simulink library "PhdLibrary"  (R2020a)
settings: Solver=VariableStepAuto  StartTime=0.0  StopTime=10.0  RelTol=1e-3
undefined symbols (not defined in the file): A1, A2, Asigma, Atilde1, Atilde2, B, B1, B2, bsigma, C1, CiL, Cmatrix, Csigma, Ctilde1, Dtilde1, Dtilde2, F1, G1, L, L1, LobsiL, magnitude, Masigma, Nasigma, ObsEp, obsSys, P2, R, R1, rho, RMSfrequency, Ro, Smep, T, ueq, x_e, xe
libraries: $bdroot x6, simulink x2, powerlib_meascontrol x1, dspstat3 x1, dspmathops x1
settings Model: Creator=d13go  LastModifiedBy=d13go

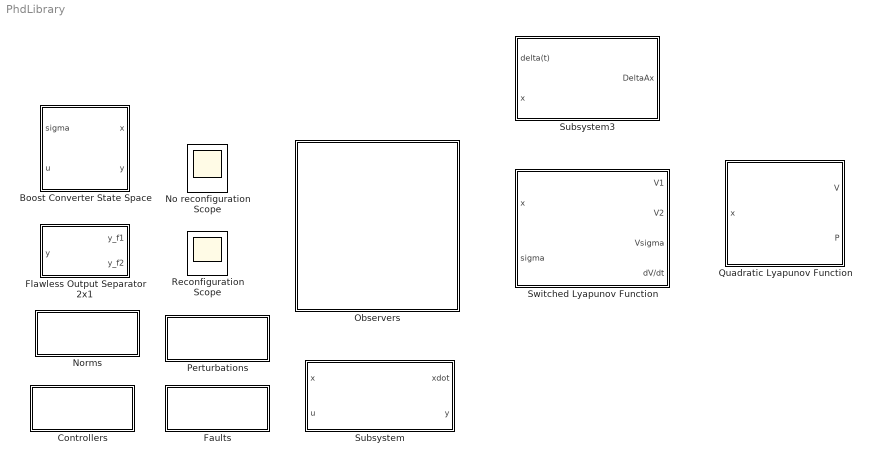
== system PhdLibrary ==
  Boost Converter State Space : Subsystem  mask(Boots State-Space model){A1=A1, A2=A2, B1=B1, R=R, Ro=Ro, Cmatrix=Cmatrix}
      mask prompts: A1 "A1 matrix"; A2 "A2 matrix"; B1 "B matrix"; R "Resistance"; Ro "Output Resistance"; Cmatrix "Output Matrix"
      mask help: Boots State-Space model
      mask Display: disp('Boost')
  Controllers : Subsystem
  Faults : Subsystem
  Flawless Output Separator 2x1 : Subsystem  mask(Flawless Output Separator){Cf1=0, Cf2=0}
      mask prompts: Cf1 "Fault matrix 1"; Cf2 "Fault matrix 2"
      mask help: Separates the 2x1 output
  No reconfiguration Scope : Scope
  Norms : Subsystem
  Observers : Subsystem
  Perturbations : Subsystem
  Quadratic Lyapunov Function : Subsystem  mask{P=P2}
      mask DialogControl DescTextVar Prompt: V = x'Px
      mask Display: disp('Quadratic \nLyapunov \nfunction')
  Reconfiguration Scope : Scope
  Subsystem : Subsystem  mask{A=A1, B=B1, C=C1}
      mask prompts: A "Matrix A"; B "Matrix B"; C "Matrix C"
      mask Display: disp('Static State Space \n xdot = Ax+Bu\n y =Cx')
  Subsystem3 : Subsystem  mask{M=Masigma{1}, N=Nasigma{1}}
      mask prompts: M "M matrix"; N "N matrix"
      mask DialogControl DescTextVar Prompt: Uncertainties matrices of type \DeltaA = delta(t)*MaNa*x(t)
      mask Display: disp('Norm-bounded \n uncertainty')
  Switched Lyapunov Function : Subsystem  mask{P1=obsSys{3}.P{1}, P2=obsSys{3}.P{2}}
      mask Display: disp('Switched \n Lyapunov \n Function\n 2-Subsystems')

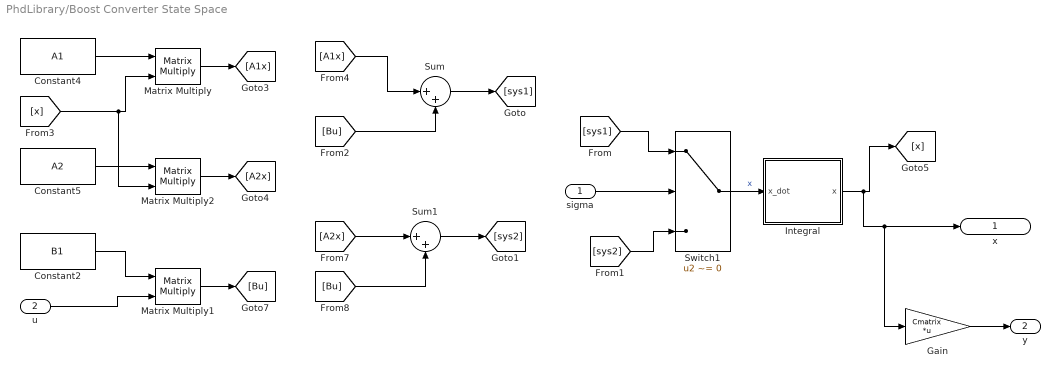
== system PhdLibrary/Boost Converter State Space ==
  sigma : Inport
  u : Inport  Port=2
  Constant2 : Constant  Value=B1  VectorParams1D=off
  Constant4 : Constant  Value=A1  VectorParams1D=off
  Constant5 : Constant  Value=A2  VectorParams1D=off
  Gain : Gain  Gain=Cmatrix  Multiplication=Matrix(K*u)
  Integral : Subsystem
  Matrix Multiply : Product  Multiplication=Matrix(*)
  Matrix Multiply1 : Product  Multiplication=Matrix(*)
  Matrix Multiply2 : Product  Multiplication=Matrix(*)
  Sum : Sum  Inputs=|++
  Sum1 : Sum  Inputs=|++
  Switch1 : Switch  Criteria=u2 ~= 0
  x : Outport
  y : Outport  Port=2
  wires:
  [A1x] -> Sum/1
  [x] -> Matrix Multiply2/2, Matrix Multiply/2
  [Bu] -> Sum1/2
  [Bu] -> Sum/2
  Constant5/1 -> Matrix Multiply2/1
  Constant4/1 -> Matrix Multiply/1
  Matrix Multiply2/1 -> [A2x]
  [sys1] -> Switch1/1
  Matrix Multiply/1 -> [A1x]
  Sum/1 -> [sys1]
  Sum1/1 -> [sys2]
  [sys2] -> Switch1/3
  Switch1/1 -> Integral/1(x_dot)  "x"
  [A2x] -> Sum1/1
  sigma/1 -> Switch1/2
  Constant2/1 -> Matrix Multiply1/1
  Matrix Multiply1/1 -> [Bu]
  u/1 -> Matrix Multiply1/2
  Integral/1(x) -> Gain/1, x/1, [x]
  Gain/1 -> y/1

== system PhdLibrary/Controllers ==
  Equilibrium Point : Subsystem  mask(Equilibrium point){R=0, Ro=0}
      mask prompts: R "Resistance"; Ro "Output resistance"
      mask help: Calculates the equilibrium point
  Integral Sliding Mode Controller : Subsystem  mask(Sliding mode controller){KiVc=2.3, KVc=0.2, ueq=ueq, Smep=Smep, KiL=2, Freq=7000}
      mask prompts: KiVc "Integral voltage gain"; KVc "Voltage gain"; ueq "Equilibrium signal"; Smep "Surface limit layer"; KiL "Current gain"; Freq "Frequency"
      mask help: Sliding mode controller with integral for boost converter
  Limit Layer : $bdroot/Controllers/Integral Sliding  Mode Controller/SlidingSurface  Smep=Smep
  Subsystem1 : Subsystem  mask{A=A1, B=B1}
      mask prompts: A "A matrx"; B "B matrix"
      mask Display: disp("Switching \n Signal \n 1-subsystem");
  Switched Affine Control : Subsystem  mask(Switched linear affine Controler){A1=0, A2=0, B1=0, B2=0, P=0}
      mask prompts: A1 "System matrix 1:"; A2 "System matrix 2:"; B1 "Input matrix 1:"; B2 "Input matrix 2:"; P "Gain matrix:"
      mask help: Controller to generate a switching law according to the equilibrium point xe

== system PhdLibrary/Faults ==
  Fault Detector : Subsystem  mask(Fault detector){Jth=0}
      mask prompts: Jth "Residual threshold"
      mask help: Generates alarm (1) if J > Jth
  Loss of sensor Generator : Subsystem  mask(Loss of sensor signal fault generator){}
      mask help: Loss of signal fault
  Noise Fault Generator : Subsystem  mask(Noise fault generator){}
      mask help: Generates noise in the desired sensor
  Offset Fault Generator : Subsystem  mask(Step faults){s1gain=20, s2gain=20}
      mask prompts: s1gain "Sensor 1 fault gain:"; s2gain "Sensor 2 fault gain:"
      mask help: Configure a step fault
  Sensor Gain Fault Generator : Subsystem  mask(Sensor gain fault generator){s1gain=0, s2gain=0}
      mask prompts: s1gain "Sensor 1 gain fault:"; s2gain "Sensor 2 gain fault:"
      mask help: Generates a gain fault in each sensor

== system PhdLibrary/Flawless Output Separator 2x1 ==
  y : Inport
  Matrizes A1 : Constant  Value=Cf2  VectorParams1D=off
  Matrizes A2 : Constant  Value=Cf1  VectorParams1D=off
  Product : Product  Multiplication=Matrix(*)
  Product1 : Product  Multiplication=Matrix(*)
  y_f1 : Outport
  y_f2 : Outport  Port=2
  wires:
  y/1 -> Product1/2, Product/2
  Matrizes A2/1 -> Product/1
  Matrizes A1/1 -> Product1/1
  Product/1 -> y_f1/1
  Product1/1 -> y_f2/1

== system PhdLibrary/Norms ==
  Norm : Subsystem
      mask DialogControl DescTextVar Prompt: Norm of a vector corresponding to ||u|| or \sqrt(u'u)
      mask Display: disp('Norm')
  Residual Evaluation RMS : Subsystem  mask{RMSfrequency=RMSfrequency/10}
      mask prompts: RMSfrequency "Windows length:"
      mask help: RMS generator for two dimensios

== system PhdLibrary/Observers ==
  Augmented Error Generator : Subsystem  mask{Cmatrix=Cmatrix, Ctilde1=Ctilde1}
      mask prompts: Cmatrix "Output Matrix"; Ctilde1 "Output matrix augmented:"
  FDSMOSLS : Subsystem  mask(Sliding mode observer){G=G1, F=F1, Atilde1=Atilde1, Atilde2=Atilde2, Dtilde1=Dtilde1, Dtilde2=Dtilde2, Ctilde1=Ctilde1, rho=rho}
      mask prompts: G "G matrix"; F "F matrix"; Atilde1 "A1 matrix augmented"; Atilde2 "A2 matrix augmented"; Dtilde1 "D1 matrix augmented"; Dtilde2 "D2 matrix augmented"; Ctilde1 "C1 matrix augmented"; rho "Sliding surface coefficient (rho)"
      mask help: Sligin mode observer for fault detection in switched affine linear systems
      mask Help: Enter the system matrices and the observer gains
      mask Display: disp('\dot{x} = Ax + b \\ y = Cx','texmode','on');
  ROSLSO 2 Subsystems : Subsystem  mask(ROSLSO){B1=0, B2=0, T=0, F1=0, F2=0, L1=0, L2=0, Q=0, z0=0}
      mask prompts: B1 "Input matrix system 1:"; B2 "Input matrix system 2:"; T "Input gain matrix:"; F1 "Observer matrix system 1:"; F2 "Observer matrix system 2:"; L1 "Output gain matrix system 1:"; L2 "Output gain matrix system 2:"; Q "Weight matrix"; z0 "Initial conditions:"
      mask help:
      | Reduced Order Switched Linear Systems Observer
      | Estimates only the unmensured variables and concatenate with output
  Reduced Order Observer : Subsystem  mask(Reduced order observer for linear systems){F=0, L=0, T=0, B=0, Q=0, z0=0}
      mask prompts: F "Observer gain matrix:"; L "Output gain matrix:"; T "Input gain matrix:"; B "Input matrix:"; Q "Weight matrix:"; z0 "Intial conditions"
      mask help:
      | Generates the estimation of unmeasured outputs with a concatenation of the output
      | z is the output unmeasured
      | x hat is the whole state estimation
  Reduced Order Derivate Z : Subsystem  mask(Reduced Order Observer Derivate Z){F=0, L=L, T=T, B=B}
      mask prompts: F "Observer gain matrix:"; L "Output gain matrix:"; T "Input gain matrix:"; B "Input matrix:"
      mask help: Reduced Order Observer Derivate Z generates just zdot, without feedbak
  Residual Generator : Subsystem  mask{A=A1, B=B1, L=L1, C=C1, R=R1}
      mask prompts: A "Matrix A"; B "Matrix B"; L "Matrix L"; C "Matrix C"; R "Matrix R"
      mask DialogControl DescTextVar Prompt: dxhat/dt = A*xhat + B*u + L*(y-yhat)
      mask DialogControl Control2 Prompt: yhat = C*xhat
      mask Display: disp('Luenberger Residual \n Generator')
  SMOSLS : Subsystem  mask(Sliding mode observer for Switched linear affine systems){A1=A1, A2=A2, B1=B1, B2=B2, C1=CiL, L=LobsiL, Smep=ObsEp, yhat0=0, x0=[0;0]}
      mask prompts: A1 "System matrix 1:"; A2 "System matrix 2:"; B1 "Input matrix 1:"; B2 "Input matrix 2:"; C1 "Output matrix 1:"; L "Observer gain:"; Smep "Limit layer:"; yhat0 "Output initial condition:"; x0 "Observer initial condition:"
      mask help: Full order observer that estimates the full state of a switched affine linear system
  Switched Residual Generator : Subsystem  mask(Boots State-Space model){A1=obsSys{2}.Asigma{1,1}, B1=obsSys{2}.bsigma{1,1}, L1=obsSys{2}.Lsigma{1,1}, C1=obsSys{2}.Csigma{1,1}, R1=obsSys{2}.Rsigma{1,1}, A2=obsSys{2}.Asigma{1,2}, B2=obsSys{2}.bsigma{1,1}, C2=obsSys{2}.Csigma{1,1}, L2=obsSys{2}.Lsigma{1,2}, R2=obsSys{2}.Rsigma{1,2}}
      mask prompts: A1 "A1 matrix"; B1 "B1 matrix"; L1 "L1 matrix"; C1 "C1 Matrix"; R1 "R1 matrix"; A2 "A2 matrix"; B2 "B2 matrix"; C2 "C2 matrix"; L2 "L2 matrix"; R2 "R2 matrix"
      mask help: Boots State-Space model
      mask DialogControl DescTextVar Prompt: dxhat/dt = A(sigma)*xhat+B(sigma)*u + L(sigma)*(y-yhat)
      mask DialogControl Control2 Prompt: yhat = C(sigma)*xhat
      mask DialogControl Control3 Prompt: r = R(sigma)*(y-yhat)
      mask DialogControl Subsystem1 Prompt: Subsystem 1
      mask DialogControl Subsystem2 Prompt: Subsytem 2
      mask Display: disp('Switched Luenberger \n Residual Generator \n 2-Subsystems')
  Uncertain Cuk : Subsystem  mask{A1=Asigma{1}, B1=bsigma{1}, C1=Csigma{1}, A2=Asigma{2}, B2=bsigma{2}, C2=Csigma{2}}
      mask prompts: A1 "Matrix A"; B1 "Matrix B"; C1 "Matrix C"; A2 "Matrix A"; B2 "Matrix B"; C2 "Matrix C"
      mask DialogControl DescTextVar Prompt: dx/dt = A(sigma)x+ B(sigma)u + wx(sigma,x,u,t)
      mask DialogControl Control2 Prompt: y = C(sigma)x + wy(sigma,x,u,t)
      mask DialogControl Container3 Prompt: Subsystem 1
      mask DialogControl Container4 Prompt: Subsystem 2
      mask Display: disp('Switched Perturbed State Space \n 2-Subsystems')

== system PhdLibrary/Perturbations ==
  Step Perturbation : Subsystem  mask(Step Perturbation){SignalSwitch=0, InitialMagnitude=0, InitialTime=0, Magnitude=0, Duration=0}
      mask prompts: SignalSwitch "Type of perturbation:"; InitialMagnitude "Initial magnitude"; InitialTime "Initial time:"; Duration "Duration (if transient):"
      mask help:
      | Insert a  persistent or transient step perturbation in the system with given magnitude and time.
      | Type of perturbation: 1 if persistent, 0 if transient
  Transient Step Perturbation : Subsystem  mask(Step perturbation){InitialTime=0.5, Duration=0.1, InitialMagnitude=0, Magnitude=1}
      mask prompts: InitialTime "Initial time:"; InitialMagnitude "Initial magnitude:"
      mask help: Insert a step perturbation with time delta

== system PhdLibrary/Quadratic Lyapunov Function ==
  x : Inport
  Constant : Constant  Value=P
  Gain : Gain  Gain=P  Multiplication=Matrix(u*K)
  Matrix Multiply : Product  Multiplication=Matrix(*)
  Transpose : Math  Operator=transpose  SaturateOnIntegerOverflow=on
  V : Outport
  P : Outport  Port=2
  wires:
  x/1 -> Matrix Multiply/2, Transpose/1
  Matrix Multiply/1 -> V/1
  Transpose/1 -> Gain/1
  Constant/1 -> P/1
  Gain/1 -> Matrix Multiply/1

== system PhdLibrary/Subsystem ==
  x : Inport
  u : Inport  Port=2
  Gain : Gain  Gain=B  Multiplication=Matrix(K*u) (u vector)
  Gain1 : Gain  Gain=A  Multiplication=Matrix(K*u) (u vector)
  Gain2 : Gain  Gain=C  Multiplication=Matrix(K*u) (u vector)
  Sum : Sum  Inputs=|++
  xdot : Outport
  y : Outport  Port=2
  wires:
  u/1 -> Gain/1
  x/1 -> Gain2/1, Gain1/1
  Gain1/1 -> Sum/1
  Gain/1 -> Sum/2
  Sum/1 -> xdot/1
  Gain2/1 -> y/1

== system PhdLibrary/Subsystem3 ==
  delta(t) : Inport
  x : Inport  Port=2
  Constant : Constant  Value=M
  Constant1 : Constant  Value=N
  Matrix Multiply1 : Product
  Matrix Multiply2 : Product  Multiplication=Matrix(*)
  Matrix Multiply3 : Product  Multiplication=Matrix(*)
  DeltaAx : Outport
  wires:
  Constant/1 -> Matrix Multiply3/1
  Constant1/1 -> Matrix Multiply3/2
  Matrix Multiply3/1 -> Matrix Multiply1/2
  delta(t)/1 -> Matrix Multiply1/1
  Matrix Multiply1/1 -> Matrix Multiply2/1
  x/1 -> Matrix Multiply2/2
  Matrix Multiply2/1 -> DeltaAx/1

== system PhdLibrary/Switched Lyapunov Function ==
  x : Inport
  sigma : Inport  Port=2
  Derivative : Derivative
  Quadratic Lyapunov Function2 : $bdroot/Quadratic Lyapunov Function  P=P2
  Quadratic Lyapunov Function3 : $bdroot/Quadratic Lyapunov Function  P=P2
  Switch : Switch  Threshold=2
  V1 : Outport
  V2 : Outport  Port=2
  Vsigma : Outport  Port=3
  dV/dt : Outport  Port=4
  wires:
  Quadratic Lyapunov Function3/1 -> Switch/1, V2/1
  Quadratic Lyapunov Function2/1 -> Switch/3, V1/1
  x/1 -> Quadratic Lyapunov Function3/1, Quadratic Lyapunov Function2/1
  sigma/1 -> Switch/2
  Switch/1 -> Derivative/1, Vsigma/1
  Derivative/1 -> dV/dt/1

== system PhdLibrary/Boost Converter State Space/Integral ==
  x_dot : Inport
  Ground : Ground
  Ground1 : Ground
  IC : InitialCondition  Value=[0;0]
  Integrator1 : Integrator  InitialConditionSource=external  InitialCondition=[-x_e; 0; 0]
  Mux : Mux  Inputs=2
  x : Outport
  wires:
  x_dot/1 -> Integrator1/1
  Integrator1/1 -> x/1
  IC/1 -> Integrator1/2
  Ground1/1 -> Mux/2
  Ground/1 -> Mux/1
  Mux/1 -> IC/1

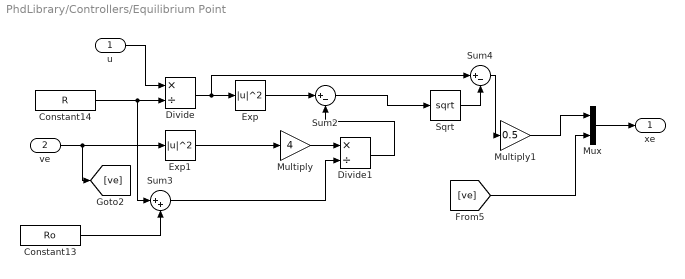
== system PhdLibrary/Controllers/Equilibrium Point ==
  u : Inport
  ve : Inport  Port=2
  Constant13 : Constant  Value=Ro  VectorParams1D=off
  Constant14 : Constant  Value=R  VectorParams1D=off
  Divide : Product  Inputs=*/
  Divide1 : Product  Inputs=*/
  Exp : Math  Operator=magnitude^2  SaturateOnIntegerOverflow=on
  Exp1 : Math  Operator=magnitude^2  SaturateOnIntegerOverflow=on
  Multiply : Gain  Gain=4
  Multiply1 : Gain  Gain=0.5
  Mux : Mux  Inputs=2
  Sqrt : Sqrt  SaturateOnIntegerOverflow=on
  Sum2 : Sum  Inputs=|+-
  Sum3 : Sum  Inputs=|++
  Sum4 : Sum  Inputs=|+-
  xe : Outport
  wires:
  Divide/1 -> Sum4/1, Exp/1
  Sum3/1 -> Divide1/2
  Sum4/1 -> Multiply1/1
  [ve] -> Mux/2
  Multiply/1 -> Divide1/1
  u/1 -> Divide/1
  Constant13/1 -> Sum3/2
  Sqrt/1 -> Sum4/2
  ve/1 -> [ve], Exp1/1
  Exp/1 -> Sum2/1
  Multiply1/1 -> Mux/1
  Mux/1 -> xe/1
  Sum2/1 -> Sqrt/1
  Constant14/1 -> Sum3/1, Divide/2
  Divide1/1 -> Sum2/2
  Exp1/1 -> Multiply/1

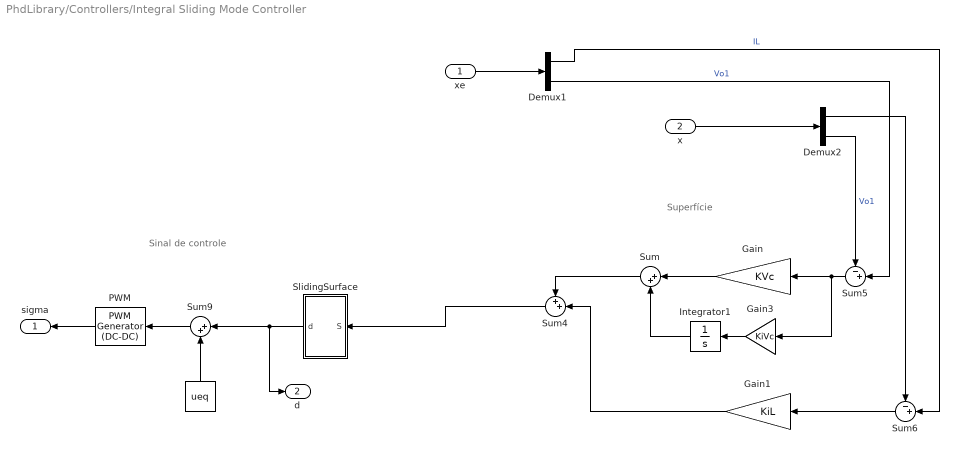
== system PhdLibrary/Controllers/Integral Sliding Mode Controller ==
  note: Sinal de controle
  note: Superfície
  xe : Inport
  x : Inport  Port=2
  "    " : Constant  Value=ueq
  Demux1 : Demux  Outputs=2
  Demux2 : Demux  Outputs=2
  Gain : Gain  Gain=KVc
  Gain1 : Gain  Gain=KiL
  Gain3 : Gain  Gain=KiVc
  Integrator1 : Integrator
  PWM : powerlib_meascontrol/Pulse & Signal Generators/PWM Generator (DC-DC)  Fsw=Freq  Ts=0
  SlidingSurface : Subsystem  mask(Sliding mode limit layer){Smep=Smep}
      mask prompts: Smep "Limit layer value"
      mask help: Define a limit layer for the sliding mode signal
      mask DialogControl ParametersGroupVar Prompt: Parameters
  Sum : Sum  Inputs=|++
  Sum4 : Sum  Inputs=++|
  Sum5 : Sum  Inputs=-+|
  Sum6 : Sum  Inputs=-+|
  Sum9 : Sum  Inputs=|++
  sigma : Outport
  d : Outport  Port=2
  wires:
  Demux1/1 -> Sum6/2  "IL"
  PWM/1 -> sigma/1
  Demux2/2 -> Sum5/1  "Vo1"
  "    "/1 -> Sum9/2
  Sum5/1 -> Gain3/1, Gain/1
  Sum9/1 -> PWM/1
  Demux1/2 -> Sum5/2  "Vo1"
  Demux2/1 -> Sum6/1
  x/1 -> Demux2/1
  Gain1/1 -> Sum4/2
  Gain/1 -> Sum/1
  Sum/1 -> Sum4/1
  SlidingSurface/1(d) -> d/1, Sum9/1
  Sum6/1 -> Gain1/1
  Gain3/1 -> Integrator1/1
  Sum4/1 -> SlidingSurface/1(S)
  Integrator1/1 -> Sum/2
  xe/1 -> Demux1/1

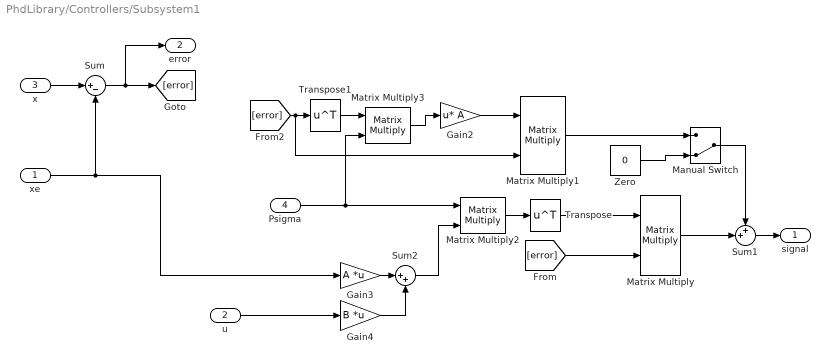
== system PhdLibrary/Controllers/Subsystem1 ==
  xe : Inport
  u : Inport  Port=2
  x : Inport  Port=3
  Psigma : Inport  Port=4
  Gain2 : Gain  Gain=A  Multiplication=Matrix(u*K)
  Gain3 : Gain  Gain=A  Multiplication=Matrix(K*u)
  Gain4 : Gain  Gain=B  Multiplication=Matrix(K*u)
  Manual Switch : ManualSwitch  CurrentSetting=0
  Matrix Multiply{,1..3} (4 alike) : Product  Multiplication=Matrix(*)
  Sum : Sum  Inputs=|+-
  Sum1 : Sum  Inputs=++|
  Sum2 : Sum  Inputs=|++
  Transpose : Math  Operator=transpose  SaturateOnIntegerOverflow=on
  Transpose1 : Math  Operator=transpose  SaturateOnIntegerOverflow=on
  Zero : Constant  Value=0  OutDataTypeStr=Inherit: Inherit via back propagation
  signal : Outport
  error : Outport  Port=2
  wires:
  Matrix Multiply2/1 -> Transpose/1
  Gain3/1 -> Sum2/1
  u/1 -> Gain4/1
  Gain4/1 -> Sum2/2
  x/1 -> Sum/1
  Sum/1 -> error/1, [error]
  [error] -> Matrix Multiply/2
  Transpose/1 -> Matrix Multiply/1
  Matrix Multiply/1 -> Sum1/2
  Sum1/1 -> signal/1
  Gain2/1 -> Matrix Multiply1/1
  [error] -> Matrix Multiply1/2, Transpose1/1
  xe/1 -> Sum/2, Gain3/1
  Psigma/1 -> Matrix Multiply3/2, Matrix Multiply2/1
  Matrix Multiply3/1 -> Gain2/1
  Transpose1/1 -> Matrix Multiply3/1
  Sum2/1 -> Matrix Multiply2/2
  Matrix Multiply1/1 -> Manual Switch/1
  Manual Switch/1 -> Sum1/1
  Zero/1 -> Manual Switch/2

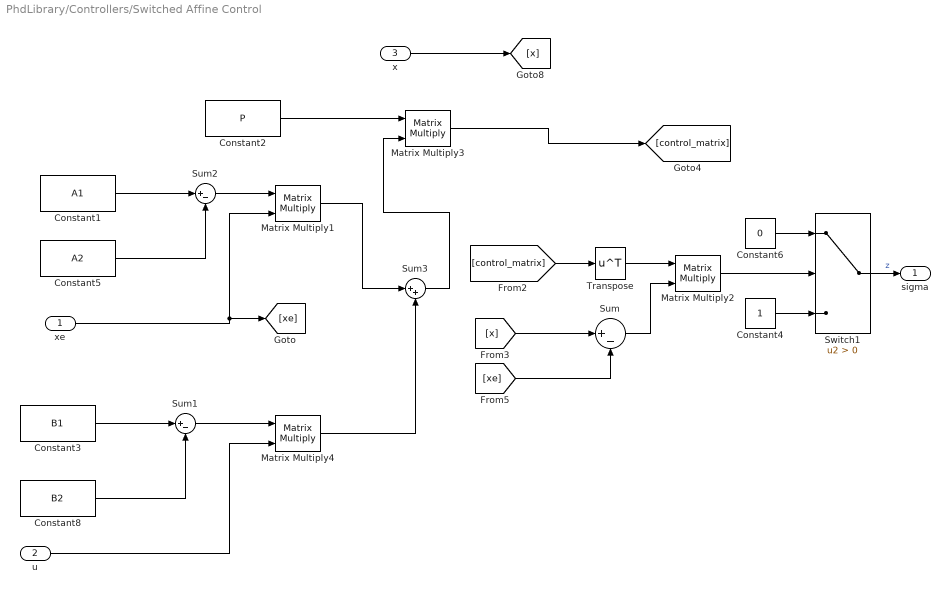
== system PhdLibrary/Controllers/Switched Affine Control ==
  xe : Inport
  u : Inport  Port=2
  x : Inport  Port=3
  Constant1 : Constant  Value=A1  VectorParams1D=off
  Constant2 : Constant  Value=P  VectorParams1D=off
  Constant3 : Constant  Value=B1  VectorParams1D=off
  Constant4 : Constant
  Constant5 : Constant  Value=A2  VectorParams1D=off
  Constant6 : Constant  Value=0
  Constant8 : Constant  Value=B2  VectorParams1D=off
  Matrix Multiply{1..4} (4 alike) : Product  Multiplication=Matrix(*)
  Sum : Sum  Inputs=|+-
  Sum1 : Sum  Inputs=|+-
  Sum2 : Sum  Inputs=|+-
  Sum3 : Sum  Inputs=|++
  Switch1 : Switch  Criteria=u2 > Threshold
  Transpose : Math  Operator=transpose  SaturateOnIntegerOverflow=on
  sigma : Outport
  wires:
  Constant5/1 -> Sum2/2
  Matrix Multiply2/1 -> Switch1/2
  [control_matrix] -> Transpose/1
  Constant1/1 -> Sum2/1
  Constant6/1 -> Switch1/1
  Sum/1 -> Matrix Multiply2/2
  [xe] -> Sum/2
  [x] -> Sum/1
  Constant4/1 -> Switch1/3
  x/1 -> [x]
  Transpose/1 -> Matrix Multiply2/1
  Constant2/1 -> Matrix Multiply3/1
  Switch1/1 -> sigma/1  "z"
  Constant3/1 -> Sum1/1
  Constant8/1 -> Sum1/2
  Sum2/1 -> Matrix Multiply1/1
  Sum1/1 -> Matrix Multiply4/1
  u/1 -> Matrix Multiply4/2
  xe/1 -> [xe], Matrix Multiply1/2
  Matrix Multiply1/1 -> Sum3/1
  Matrix Multiply4/1 -> Sum3/2
  Sum3/1 -> Matrix Multiply3/2
  Matrix Multiply3/1 -> [control_matrix]

== system PhdLibrary/Faults/Fault Detector ==
  Residual : Inport
  Constant10 : Constant
  Constant9 : Constant  Value=0
  Fault Detecition : Switch  Criteria=u2 > Threshold  Threshold=Jth  ZeroCross=off
  Alarm : Outport
  wires:
  Constant9/1 -> Fault Detecition/3
  Constant10/1 -> Fault Detecition/1
  Fault Detecition/1 -> Alarm/1
  Residual/1 -> Fault Detecition/2

== system PhdLibrary/Faults/Loss of sensor Generator ==
  y : Inport
  faultType : Inport  Port=2
  Constant4 : Constant  Value=[1 0;0 1]  VectorParams1D=off
  Constant7 : Constant  Value=[0 0;0 1]  VectorParams1D=off
  Constant8 : Constant  Value=[1 0;0 0]  VectorParams1D=off
  Fault Switch : MultiPortSwitch  DataPortOrder=Zero-based contiguous  DataPortForDefault=Additional data port  zeroidx=on
  Matrix Multiply : Product  Multiplication=Matrix(*)
  yfault : Outport
  wires:
  Constant7/1 -> Fault Switch/3
  Constant4/1 -> Fault Switch/5, Fault Switch/2
  Constant8/1 -> Fault Switch/4
  Fault Switch/1 -> Matrix Multiply/1
  faultType/1 -> Fault Switch/1
  Matrix Multiply/1 -> yfault/1
  y/1 -> Matrix Multiply/2

== system PhdLibrary/Faults/Noise Fault Generator ==
  y : Inport
  faultType : Inport  Port=2
  Band-Limited White Noise1 : simulink/Sources/Band-Limited White Noise  Cov=[0.1]  Ts=0.1  seed=[23341]  VectorParams1D=off
  Constant2 : Constant  Value=[0 0;0 0]  VectorParams1D=off
  Constant5 : Constant  Value=[1 0;0 0]  VectorParams1D=off
  Constant6 : Constant  Value=[0 0;0 1]  VectorParams1D=off
  Matrix Multiply : Product  Multiplication=Matrix(*)
  Noise Fault Switch : MultiPortSwitch  DataPortOrder=Zero-based contiguous  DataPortForDefault=Additional data port  zeroidx=on
  Sum1 : Sum  Inputs=|++
  yfault : Outport
  wires:
  faultType/1 -> Noise Fault Switch/1
  Constant5/1 -> Noise Fault Switch/3
  Constant6/1 -> Noise Fault Switch/4
  Band-Limited White Noise1/1 -> Matrix Multiply/2
  Noise Fault Switch/1 -> Matrix Multiply/1
  Constant2/1 -> Noise Fault Switch/5, Noise Fault Switch/2
  Sum1/1 -> yfault/1
  y/1 -> Sum1/2
  Matrix Multiply/1 -> Sum1/1

== system PhdLibrary/Faults/Offset Fault Generator ==
  y : Inport
  faultType : Inport  Port=2
  Constant4 : Constant  Value=[s1gain;0]  VectorParams1D=off
  Constant7 : Constant  Value=[0;s2gain]  VectorParams1D=off
  Constant8 : Constant  Value=[0;0]  VectorParams1D=off
  Sum : Sum  Inputs=|++
  iLFault Switch : MultiPortSwitch  DataPortOrder=Zero-based contiguous  DataPortForDefault=Additional data port  zeroidx=on
  y_fault : Outport
  wires:
  y/1 -> Sum/2
  Constant8/1 -> iLFault Switch/5, iLFault Switch/2
  iLFault Switch/1 -> Sum/1
  Constant7/1 -> iLFault Switch/4
  Constant4/1 -> iLFault Switch/3
  faultType/1 -> iLFault Switch/1
  Sum/1 -> y_fault/1

== system PhdLibrary/Faults/Sensor Gain Fault Generator ==
  y : Inport
  faultType : Inport  Port=2
  Constant4 : Constant  Value=[1 0;0 1]  VectorParams1D=off
  Constant7 : Constant  Value=[s1gain 0;0 1]  VectorParams1D=off
  Constant8 : Constant  Value=[1 0;0 s2gain]  VectorParams1D=off
  Matrix Multiply : Product  Multiplication=Matrix(*)
  iLFault Switch : MultiPortSwitch  DataPortOrder=Zero-based contiguous  DataPortForDefault=Additional data port  zeroidx=on
  yfault : Outport
  wires:
  Matrix Multiply/1 -> yfault/1
  faultType/1 -> iLFault Switch/1
  Constant8/1 -> iLFault Switch/4
  iLFault Switch/1 -> Matrix Multiply/1
  Constant7/1 -> iLFault Switch/3
  Constant4/1 -> iLFault Switch/5, iLFault Switch/2
  y/1 -> Matrix Multiply/2

== system PhdLibrary/Norms/Norm ==
  u : Inport
  Nom : MATLAB Function  TreatAsAtomicUnit=on
  ||u|| : Outport
  wires:
  Nom/1(y) -> ||u||/1
  u/1 -> Nom/1(u)

== system PhdLibrary/Norms/Residual Evaluation RMS ==
  e_y : Inport
  Moving RMS : dspstat3/Moving RMS  Method=Sliding window  ForgettingFactorPort=off  SpecifyWindowLength=on  WindowLength=RMSfrequency/10  ForgettingFactor=0.9  SimulateUsing=Code generation
      settings: SourceProductBaseCode=DS
  Subsystem6 : $bdroot/Subsystem6
  RMS : Outport
  wires:
  Subsystem6/1 -> Moving RMS/1
  Moving RMS/1 -> RMS/1
  e_y/1 -> Subsystem6/1

== system PhdLibrary/Observers/Augmented Error Generator ==
  y_fault : Inport
  xe : Inport  Port=2
  Gain1 : Gain  Gain=Cmatrix  Multiplication=Matrix(K*u)
  Gain2 : Gain  Gain=Ctilde1  Multiplication=Matrix(K*u)
  Mux : Mux  Inputs=2
  Sum4 : Sum  Inputs=-+|
  z1 : Subsystem
  e_tilde : Outport
  y_e_tilde : Outport  Port=2
  wires:
  z1/1(z) -> Mux/2
  Mux/1 -> Gain2/1, e_tilde/1
  Gain2/1 -> y_e_tilde/1
  xe/1 -> Gain1/1
  Gain1/1 -> Sum4/1
  y_fault/1 -> Sum4/2
  Sum4/1 -> Mux/1, z1/1(z_dot)

== system PhdLibrary/Observers/FDSMOSLS ==
  y_e_tilde : Inport
  sigma : Inport  Port=2
  ErrorGenerator : Subsystem
  IC2 : InitialCondition  Value=[0;0]
  Sliding Mode Observer 5 : Subsystem
  e_y : Outport
  v : Outport  Port=2
  wires:
  sigma/1 -> Sliding Mode Observer 5/3(sigma)
  y_e_tilde/1 -> ErrorGenerator/1(y_e_tilde)
  IC2/1 -> ErrorGenerator/2(y_e_tilde_hat)
  ErrorGenerator/1(e_y) -> Sliding Mode Observer 5/1(ey)
  ErrorGenerator/2(v) -> Sliding Mode Observer 5/2(v), v/1
  Sliding Mode Observer 5/2(y_e_tilde_hat) -> IC2/1
  Sliding Mode Observer 5/1(ey_out) -> e_y/1

== system PhdLibrary/Observers/ROSLSO 2 Subsystems ==
  u : Inport
  y : Inport  Port=2
  sigma : Inport  Port=3
  Constant8 : Constant  Value=Q  VectorParams1D=off
  Integrator1 : Integrator  InitialCondition=z0
  Matrix Multiply6 : Product  Multiplication=Matrix(*)
  Mux : Mux  Inputs=2
  Reduced Order Derivate Z : Subsystem  mask(Reduced Order Observer Derivate Z){F=F1, L=L1, T=T, B=B1}
      mask prompts: F "Observer gain matrix:"; L "Output gain matrix:"; T "Input gain matrix:"; B "Input matrix:"
      mask help: Reduced Order Observer Derivate Z generates just zdot, without feedbak
  Reduced Order Derivate Z1 : Subsystem  mask(Reduced Order Observer Derivate Z){F=F2, L=L2, T=T, B=B2}
      mask prompts: F "Observer gain matrix:"; L "Output gain matrix:"; T "Input gain matrix:"; B "Input matrix:"
      mask help: Reduced Order Observer Derivate Z generates just zdot, without feedbak
  Switch1 : Switch  Criteria=u2 ~= 0
  z : Outport
  xhat : Outport  Port=2
  wires:
  sigma/1 -> Switch1/2
  Switch1/1 -> Integrator1/1  "zdot"
  y/1 -> [y]
  Constant8/1 -> Matrix Multiply6/1
  Matrix Multiply6/1 -> xhat/1
  Mux/1 -> Matrix Multiply6/2
  [y] -> Mux/1
  Reduced Order Derivate Z/1(zdot) -> Switch1/1
  u/1 -> Reduced Order Derivate Z1/1(u), Reduced Order Derivate Z/1(u)
  [y] -> Reduced Order Derivate Z1/2(y), Reduced Order Derivate Z/2(y)
  [z] -> Reduced Order Derivate Z/3(z), Reduced Order Derivate Z1/3(z)
  Reduced Order Derivate Z1/1(zdot) -> Switch1/3
  Integrator1/1 -> z/1, Mux/2, [z]

== system PhdLibrary/Observers/Reduced Order Observer ==
  u : Inport
  y : Inport  Port=2
  Constant8 : Constant  Value=Q  VectorParams1D=off
  Ground : Ground
  IC : InitialCondition  Value=z0
  Integrator1 : Integrator  InitialConditionSource=external  InitialCondition=[-x_e; 0; 0]
  Matrix Multiply6 : Product  Multiplication=Matrix(*)
  Mux : Mux  Inputs=2
  Reduced Order Derivate Z : Subsystem  mask(Reduced Order Observer Derivate Z){F=0, L=L, T=T, B=B}
      mask prompts: F "Observer gain matrix:"; L "Output gain matrix:"; T "Input gain matrix:"; B "Input matrix:"
      mask help: Reduced Order Observer Derivate Z generates just zdot, without feedbak
  z : Outport
  xhat : Outport  Port=2
  wires:
  Mux/1 -> Matrix Multiply6/2
  Matrix Multiply6/1 -> xhat/1
  [y] -> Mux/1
  Constant8/1 -> Matrix Multiply6/1
  IC/1 -> Integrator1/2
  Ground/1 -> IC/1
  u/1 -> Reduced Order Derivate Z/1(u)
  Reduced Order Derivate Z/1(zdot) -> Integrator1/1
  Integrator1/1 -> Mux/2, Reduced Order Derivate Z/3(z), z/1
  y/1 -> [y], Reduced Order Derivate Z/2(y)

== system PhdLibrary/Observers/Reduced Order Derivate Z ==
  u : Inport
  y : Inport  Port=2
  z : Inport  Port=3
  Constant : Constant  Value=F  VectorParams1D=off
  Constant1 : Constant  Value=T  VectorParams1D=off
  Constant2 : Constant  Value=L  VectorParams1D=off
  Matrix Multiply{1..3,8} (4 alike) : Product  Multiplication=Matrix(*)
  MatrizesA8 : Constant  Value=B  VectorParams1D=off
  Sum : Sum  Inputs=|+++
  zdot : Outport
  wires:
  MatrizesA8/1 -> Matrix Multiply8/1
  Constant1/1 -> Matrix Multiply1/1
  z/1 -> Matrix Multiply3/2
  Matrix Multiply3/1 -> Sum/2
  Constant/1 -> Matrix Multiply3/1
  Matrix Multiply8/1 -> Matrix Multiply1/2
  Matrix Multiply1/1 -> Sum/1
  u/1 -> Matrix Multiply8/2
  Sum/1 -> zdot/1
  Constant2/1 -> Matrix Multiply2/1
  Matrix Multiply2/1 -> Sum/3
  y/1 -> Matrix Multiply2/2

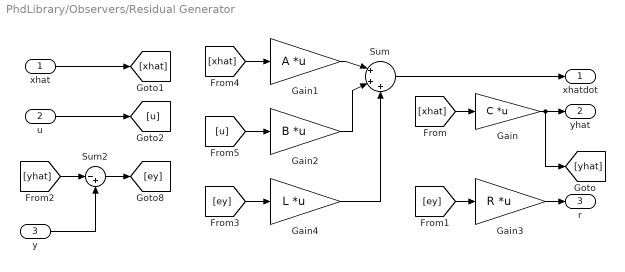
== system PhdLibrary/Observers/Residual Generator ==
  xhat : Inport
  u : Inport  Port=2
  y : Inport  Port=3
  Gain : Gain  Gain=C  Multiplication=Matrix(K*u) (u vector)
  Gain1 : Gain  Gain=A  Multiplication=Matrix(K*u) (u vector)
  Gain2 : Gain  Gain=B  Multiplication=Matrix(K*u) (u vector)
  Gain3 : Gain  Gain=R  Multiplication=Matrix(K*u) (u vector)
  Gain4 : Gain  Gain=L  Multiplication=Matrix(K*u) (u vector)
  Sum : Sum  Inputs=|+++
  Sum2 : Sum  Inputs=|-+
  xhatdot : Outport
  yhat : Outport  Port=2
  r : Outport  Port=3
  wires:
  Sum2/1 -> [ey]
  [yhat] -> Sum2/1
  y/1 -> Sum2/2
  Sum/1 -> xhatdot/1
  Gain/1 -> yhat/1, [yhat]
  xhat/1 -> [xhat]
  [xhat] -> Gain/1
  [ey] -> Gain3/1
  Gain3/1 -> r/1
  u/1 -> [u]
  [xhat] -> Gain1/1
  Gain1/1 -> Sum/1
  [u] -> Gain2/1
  Gain2/1 -> Sum/2
  Gain4/1 -> Sum/3
  [ey] -> Gain4/1

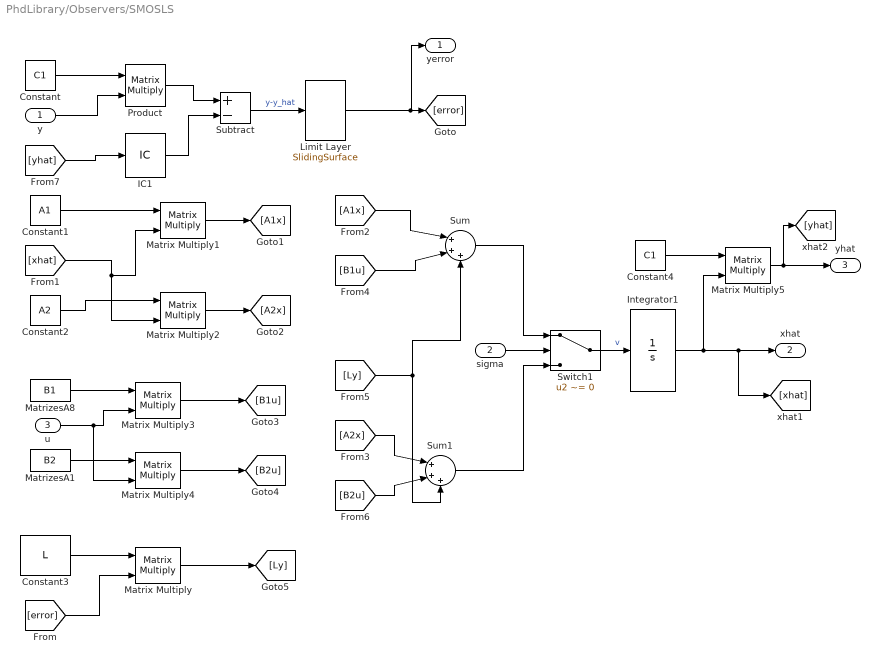
== system PhdLibrary/Observers/SMOSLS ==
  y : Inport
  sigma : Inport  Port=2
  u : Inport  Port=3
  Constant : Constant  Value=C1  VectorParams1D=off
  Constant1 : Constant  Value=A1  VectorParams1D=off
  Constant2 : Constant  Value=A2  VectorParams1D=off
  Constant3 : Constant  Value=L  VectorParams1D=off
  Constant4 : Constant  Value=C1  VectorParams1D=off
  IC1 : InitialCondition  Value=yhat0
  Integrator1 : Integrator  InitialCondition=x0
  Limit Layer : $bdroot/Integral Sliding  Mode Controller/SlidingSurface  Smep=ObsEp
  Matrix Multiply{,1..5} (6 alike) : Product  Multiplication=Matrix(*)
  MatrizesA1 : Constant  Value=B2  VectorParams1D=off
  MatrizesA8 : Constant  Value=B1  VectorParams1D=off
  Product : Product  Multiplication=Matrix(*)
  Subtract : Sum  Inputs=+-
  Sum : Sum  Inputs=|+++
  Sum1 : Sum  Inputs=|+++
  Switch1 : Switch  Criteria=u2 ~= 0
  yerror : Outport
  xhat : Outport  Port=2
  yhat : Outport  Port=3
  wires:
  Subtract/1 -> Limit Layer/1  "y-y_hat"
  Product/1 -> Subtract/1
  Limit Layer/1 -> yerror/1, [error]
  [yhat] -> IC1/1
  y/1 -> Product/2
  Constant/1 -> Product/1
  Constant3/1 -> Matrix Multiply/1
  MatrizesA8/1 -> Matrix Multiply3/1
  Sum/1 -> Switch1/1
  [error] -> Matrix Multiply/2
  Constant1/1 -> Matrix Multiply1/1
  [B1u] -> Sum/2
  Matrix Multiply4/1 -> [B2u]
  [Ly] -> Sum/3, Sum1/3
  [A2x] -> Sum1/1
  [A1x] -> Sum/1
  [B2u] -> Sum1/2
  Matrix Multiply3/1 -> [B1u]
  u/1 -> Matrix Multiply4/2, Matrix Multiply3/2
  MatrizesA1/1 -> Matrix Multiply4/1
  sigma/1 -> Switch1/2
  Matrix Multiply1/1 -> [A1x]
  Sum1/1 -> Switch1/3
  Constant4/1 -> Matrix Multiply5/1
  Constant2/1 -> Matrix Multiply2/1
  Integrator1/1 -> xhat/1, [xhat], Matrix Multiply5/2
  Matrix Multiply5/1 -> [yhat], yhat/1
  Matrix Multiply2/1 -> [A2x]
  Switch1/1 -> Integrator1/1  "v"
  Matrix Multiply/1 -> [Ly]
  [xhat] -> Matrix Multiply2/2, Matrix Multiply1/2
  IC1/1 -> Subtract/2

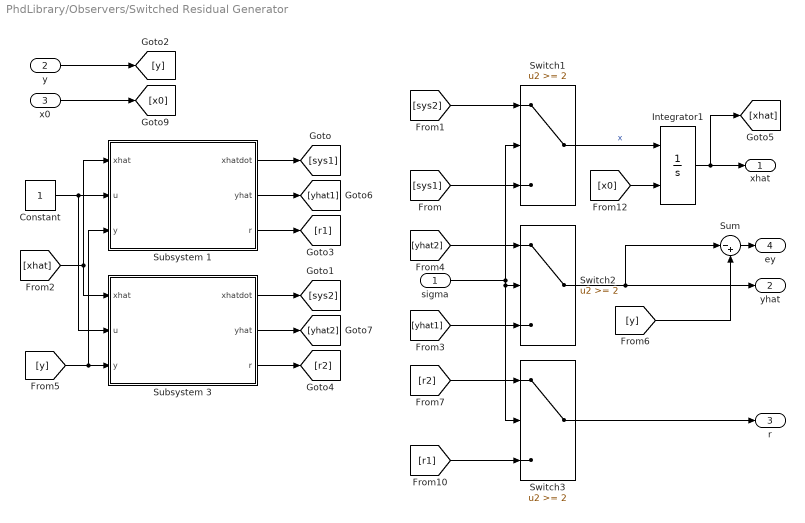
== system PhdLibrary/Observers/Switched Residual Generator ==
  sigma : Inport
  y : Inport  Port=2
  x0 : Inport  Port=3
  Constant : Constant
  Integrator1 : Integrator  InitialConditionSource=external  InitialCondition=[-x_e; 0; 0]
  Subsystem 1 : Subsystem  mask{A=A1, B=B1, L=L1, C=C1, R=R1}
      mask prompts: A "Matrix A"; B "Matrix B"; L "Matrix L"; C "Matrix C"; R "Matrix R"
      mask DialogControl DescTextVar Prompt: dxhat/dt = A*xhat + B*u + L*(y-yhat)
      mask DialogControl Control2 Prompt: yhat = C*xhat
      mask Display: disp('Luenberger Residual \n Generator')
  Subsystem 3 : Subsystem  mask{A=A2, B=B2, L=L2, C=C2, R=R2}
      mask prompts: A "Matrix A"; B "Matrix B"; L "Matrix L"; C "Matrix C"; R "Matrix R"
      mask DialogControl DescTextVar Prompt: dxhat/dt = A*xhat + B*u + L*(y-yhat)
      mask DialogControl Control2 Prompt: yhat = C*xhat
      mask Display: disp('Luenberger Residual \n Generator')
  Sum : Sum  Inputs=|-+
  Switch1 : Switch  Threshold=2
  Switch2 : Switch  Threshold=2
  Switch3 : Switch  Threshold=2
  xhat : Outport
  yhat : Outport  Port=2
  r : Outport  Port=3
  ey : Outport  Port=4
  wires:
  sigma/1 -> Switch3/2, Switch2/2, Switch1/2
  Integrator1/1 -> xhat/1, [xhat]
  [sys2] -> Switch1/1
  [sys1] -> Switch1/3
  Switch1/1 -> Integrator1/1  "x"
  x0/1 -> [x0]
  [x0] -> Integrator1/2
  Subsystem 1/1(xhatdot) -> [sys1]
  Subsystem 3/1(xhatdot) -> [sys2]
  [xhat] -> Subsystem 3/1(xhat), Subsystem 1/1(xhat)
  Constant/1 -> Subsystem 3/2(u), Subsystem 1/2(u)
  Subsystem 1/3(r) -> [r1]
  Subsystem 3/3(r) -> [r2]
  Subsystem 1/2(yhat) -> [yhat1]
  Subsystem 3/2(yhat) -> [yhat2]
  [r2] -> Switch3/1
  [r1] -> Switch3/3
  Switch2/1 -> Sum/1, yhat/1
  Switch3/1 -> r/1
  [y] -> Subsystem 3/3(y), Subsystem 1/3(y)
  y/1 -> [y]
  Sum/1 -> ey/1
  [y] -> Sum/2
  [yhat1] -> Switch2/3
  [yhat2] -> Switch2/1

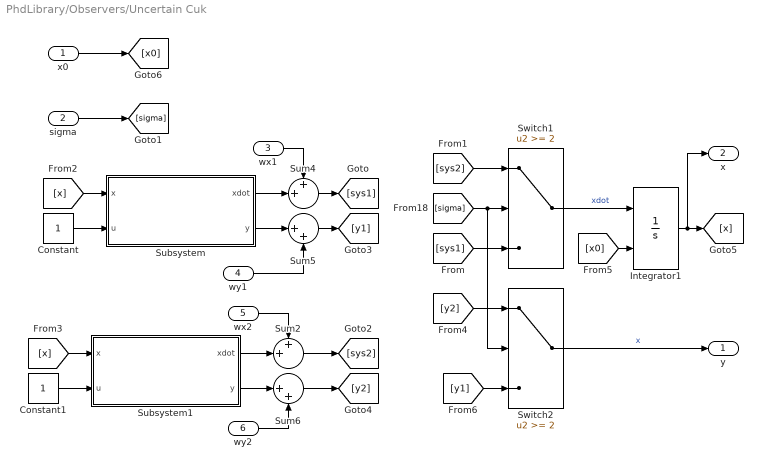
== system PhdLibrary/Observers/Uncertain Cuk ==
  x0 : Inport
  sigma : Inport  Port=2
  wx1 : Inport  Port=3
  wy1 : Inport  Port=4
  wx2 : Inport  Port=5
  wy2 : Inport  Port=6
  Constant : Constant
  Constant1 : Constant
  Integrator1 : Integrator  InitialConditionSource=external  InitialCondition=[-x_e; 0; 0]
  Subsystem : Subsystem  mask{A=A1, B=B1, C=C1}
      mask prompts: A "Matrix A"; B "Matrix B"; C "Matrix C"
      mask Display: disp('Static State Space \n xdot = Ax+Bu\n y =Cx')
  Subsystem1 : Subsystem  mask{A=A2, B=B2, C=C2}
      mask prompts: A "Matrix A"; B "Matrix B"; C "Matrix C"
      mask Display: disp('Static State Space \n xdot = Ax+Bu\n y =Cx')
  Sum2 : Sum  Inputs=++|
  Sum4 : Sum  Inputs=++|
  Sum5 : Sum  Inputs=|++
  Sum6 : Sum  Inputs=|++
  Switch1 : Switch  Threshold=2
  Switch2 : Switch  Threshold=2
  y : Outport
  x : Outport  Port=2
  wires:
  [sys2] -> Switch1/1
  [sys1] -> Switch1/3
  [sigma] -> Switch2/2, Switch1/2
  Subsystem/1(xdot) -> Sum4/2
  Subsystem/2(y) -> Sum5/1
  Sum4/1 -> [sys1]
  Sum5/1 -> [y1]
  [x] -> Subsystem/1(x)
  Constant/1 -> Subsystem/2(u)
  Switch1/1 -> Integrator1/1  "xdot"
  [x0] -> Integrator1/2
  Integrator1/1 -> x/1, [x]
  Sum6/1 -> [y2]
  Sum2/1 -> [sys2]
  Subsystem1/2(y) -> Sum6/1
  [x] -> Subsystem1/1(x)
  Subsystem1/1(xdot) -> Sum2/2
  Constant1/1 -> Subsystem1/2(u)
  [y2] -> Switch2/1
  [y1] -> Switch2/3
  Switch2/1 -> y/1  "x"
  sigma/1 -> [sigma]
  x0/1 -> [x0]
  wx1/1 -> Sum4/1
  wy1/1 -> Sum5/2
  wx2/1 -> Sum2/1
  wy2/1 -> Sum6/2

== system PhdLibrary/Perturbations/Step Perturbation ==
  Constant : Constant  Value=SignalSwitch  VectorParams1D=off
  Step3 : Step  Time=InitialTime  Before=InitialMagnitude  After=Magnitude  SampleTime=0
  Switch7 : Switch  Criteria=u2 ~= 0
  Transient Step Perturbation1 : $bdroot/Transient Step Perturbation  InitialTime=0.5  Duration=0.1  InitialMagnitude=0  Magnitude=1
  perturbation : Outport
  wires:
  Switch7/1 -> perturbation/1
  Constant/1 -> Switch7/2
  Step3/1 -> Switch7/1
  Transient Step Perturbation1/1 -> Switch7/3

== system PhdLibrary/Perturbations/Transient Step Perturbation ==
  Step1 : Step  Time=InitialTime  Before=InitialMagnitude  After=Magnitude  SampleTime=0
  Step2 : Step  Time=InitialTime+Duration  Before=InitialMagnitude  After=-Magnitude  SampleTime=0
  Sum : Sum  Inputs=|++
  Perturbation : Outport
  wires:
  Sum/1 -> Perturbation/1
  Step2/1 -> Sum/2
  Step1/1 -> Sum/1

== system PhdLibrary/Controllers/Integral Sliding Mode Controller/SlidingSurface ==
  S : Inport
  "    2" : Constant  Value=Smep
  Abs : Abs
  GreaterThan : RelationalOperator  Operator=>  OutDataTypeStr=boolean  RndMeth=Simplest
  If : If  IfExpression=u1 ~= 0
  If Action Subsystem : Subsystem  TreatAsAtomicUnit=on
  If Action Subsystem2 : Subsystem  TreatAsAtomicUnit=on
  Merge1 : Merge
  d : Outport
  wires:
  If Action Subsystem2/1(d) -> Merge1/2
  [S] -> If Action Subsystem/1(S), If Action Subsystem2/1(S)
  If/2 -> If Action Subsystem2/Action
  If/1 -> If Action Subsystem/Action
  [ep] -> If Action Subsystem2/2(ep)
  S/1 -> [S], Abs/1
  If Action Subsystem/1(d) -> Merge1/1
  Abs/1 -> GreaterThan/1
  GreaterThan/1 -> If/1
  Merge1/1 -> d/1
  "    2"/1 -> [ep], GreaterThan/2

== system PhdLibrary/Observers/Augmented Error Generator/z1 ==
  z_dot : Inport
  Constant1 : Constant  Value=[0;0]  VectorParams1D=off
  Gain2 : Gain  Gain=Cmatrix  Multiplication=Matrix(K*u) (u vector)
  Integrator6 : Integrator  InitialConditionSource=external
  z : Outport
  wires:
  Gain2/1 -> Integrator6/1
  Integrator6/1 -> z/1
  z_dot/1 -> Gain2/1
  Constant1/1 -> Integrator6/2

== system PhdLibrary/Observers/FDSMOSLS/ErrorGenerator ==
  y_e_tilde : Inport
  y_e_tilde_hat : Inport  Port=2
  AND : Logic  IconShape=distinctive  AllPortsSameDT=off  OutDataTypeStr=boolean
  Compare To Zero : simulink/Logic and Bit Operations/Compare To Zero  relop=~=  OutDataTypeStr=boolean
  Constant1 : Constant  Value=[0;0]
  Demux : Demux  Outputs=2
  If : If  IfExpression=u1 ~= 0
  If Action Subsystem : Subsystem  TreatAsAtomicUnit=on
  If Action Subsystem1 : Subsystem  TreatAsAtomicUnit=on
  Merge : Merge  InitialOutput=[0;0]
  Sum : Sum  Inputs=|+-
  e_y : Outport
  v : Outport  Port=2
  wires:
  Compare To Zero/1 -> Demux/1
  Merge/1 -> v/1
  AND/1 -> If/1
  Demux/2 -> AND/2
  Demux/1 -> AND/1
  If Action Subsystem1/1(v) -> Merge/2
  If Action Subsystem/1(v) -> Merge/1
  Constant1/1 -> If Action Subsystem1/1(e_y)
  [e_y] -> If Action Subsystem/1(e_y)
  If/2 -> If Action Subsystem1/Action
  If/1 -> If Action Subsystem/Action
  Sum/1 -> [e_y], e_y/1, Compare To Zero/1
  y_e_tilde_hat/1 -> Sum/2
  y_e_tilde/1 -> Sum/1

== system PhdLibrary/Observers/FDSMOSLS/Sliding Mode Observer 5 ==
  ey : Inport
  v : Inport  Port=2
  sigma : Inport  Port=3
  C : Constant  Value=Ctilde1
  ObserverDynamics : Subsystem
  Product : Product  Multiplication=Matrix(*)
  ey_out : Outport
  y_e_tilde_hat : Outport  Port=2
  wires:
  v/1 -> ObserverDynamics/2(v)
  ey/1 -> ObserverDynamics/1(ey), ey_out/1
  sigma/1 -> ObserverDynamics/3(sigma)
  ObserverDynamics/1(e_tilde_hat) -> Product/2
  C/1 -> Product/1
  Product/1 -> y_e_tilde_hat/1

== system PhdLibrary/Observers/ROSLSO 2 Subsystems/Reduced Order Derivate Z ==
  u : Inport
  y : Inport  Port=2
  z : Inport  Port=3
  Constant : Constant  Value=F  VectorParams1D=off
  Constant1 : Constant  Value=T  VectorParams1D=off
  Constant2 : Constant  Value=L  VectorParams1D=off
  Matrix Multiply{1..3,8} (4 alike) : Product  Multiplication=Matrix(*)
  MatrizesA8 : Constant  Value=B  VectorParams1D=off
  Sum : Sum  Inputs=|+++
  zdot : Outport
  wires:
  MatrizesA8/1 -> Matrix Multiply8/1
  Constant1/1 -> Matrix Multiply1/1
  z/1 -> Matrix Multiply3/2
  Matrix Multiply3/1 -> Sum/2
  Constant/1 -> Matrix Multiply3/1
  Matrix Multiply8/1 -> Matrix Multiply1/2
  Matrix Multiply1/1 -> Sum/1
  u/1 -> Matrix Multiply8/2
  Sum/1 -> zdot/1
  Constant2/1 -> Matrix Multiply2/1
  Matrix Multiply2/1 -> Sum/3
  y/1 -> Matrix Multiply2/2

== system PhdLibrary/Observers/ROSLSO 2 Subsystems/Reduced Order Derivate Z1 ==
  u : Inport
  y : Inport  Port=2
  z : Inport  Port=3
  Constant : Constant  Value=F  VectorParams1D=off
  Constant1 : Constant  Value=T  VectorParams1D=off
  Constant2 : Constant  Value=L  VectorParams1D=off
  Matrix Multiply{1..3,8} (4 alike) : Product  Multiplication=Matrix(*)
  MatrizesA8 : Constant  Value=B  VectorParams1D=off
  Sum : Sum  Inputs=|+++
  zdot : Outport
  wires:
  MatrizesA8/1 -> Matrix Multiply8/1
  Constant1/1 -> Matrix Multiply1/1
  z/1 -> Matrix Multiply3/2
  Matrix Multiply3/1 -> Sum/2
  Constant/1 -> Matrix Multiply3/1
  Matrix Multiply8/1 -> Matrix Multiply1/2
  Matrix Multiply1/1 -> Sum/1
  u/1 -> Matrix Multiply8/2
  Sum/1 -> zdot/1
  Constant2/1 -> Matrix Multiply2/1
  Matrix Multiply2/1 -> Sum/3
  y/1 -> Matrix Multiply2/2

== system PhdLibrary/Observers/Reduced Order Observer/Reduced Order Derivate Z ==
  u : Inport
  y : Inport  Port=2
  z : Inport  Port=3
  Constant : Constant  Value=F  VectorParams1D=off
  Constant1 : Constant  Value=T  VectorParams1D=off
  Constant2 : Constant  Value=L  VectorParams1D=off
  Matrix Multiply{1..3,8} (4 alike) : Product  Multiplication=Matrix(*)
  MatrizesA8 : Constant  Value=B  VectorParams1D=off
  Sum : Sum  Inputs=|+++
  zdot : Outport
  wires:
  MatrizesA8/1 -> Matrix Multiply8/1
  Constant1/1 -> Matrix Multiply1/1
  z/1 -> Matrix Multiply3/2
  Matrix Multiply3/1 -> Sum/2
  Constant/1 -> Matrix Multiply3/1
  Matrix Multiply8/1 -> Matrix Multiply1/2
  Matrix Multiply1/1 -> Sum/1
  u/1 -> Matrix Multiply8/2
  Sum/1 -> zdot/1
  Constant2/1 -> Matrix Multiply2/1
  Matrix Multiply2/1 -> Sum/3
  y/1 -> Matrix Multiply2/2

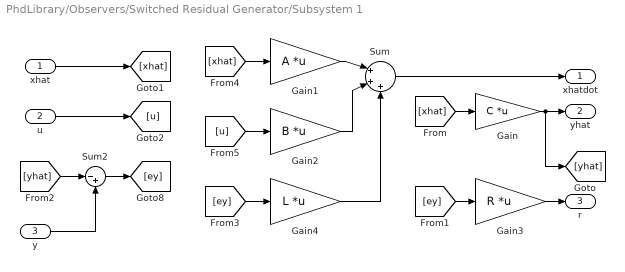
== system PhdLibrary/Observers/Switched Residual Generator/Subsystem 1 ==
  xhat : Inport
  u : Inport  Port=2
  y : Inport  Port=3
  Gain : Gain  Gain=C  Multiplication=Matrix(K*u) (u vector)
  Gain1 : Gain  Gain=A  Multiplication=Matrix(K*u) (u vector)
  Gain2 : Gain  Gain=B  Multiplication=Matrix(K*u) (u vector)
  Gain3 : Gain  Gain=R  Multiplication=Matrix(K*u) (u vector)
  Gain4 : Gain  Gain=L  Multiplication=Matrix(K*u) (u vector)
  Sum : Sum  Inputs=|+++
  Sum2 : Sum  Inputs=|-+
  xhatdot : Outport
  yhat : Outport  Port=2
  r : Outport  Port=3
  wires:
  Sum2/1 -> [ey]
  [yhat] -> Sum2/1
  y/1 -> Sum2/2
  Sum/1 -> xhatdot/1
  Gain/1 -> yhat/1, [yhat]
  xhat/1 -> [xhat]
  [xhat] -> Gain/1
  [ey] -> Gain3/1
  Gain3/1 -> r/1
  u/1 -> [u]
  [xhat] -> Gain1/1
  Gain1/1 -> Sum/1
  [u] -> Gain2/1
  Gain2/1 -> Sum/2
  Gain4/1 -> Sum/3
  [ey] -> Gain4/1

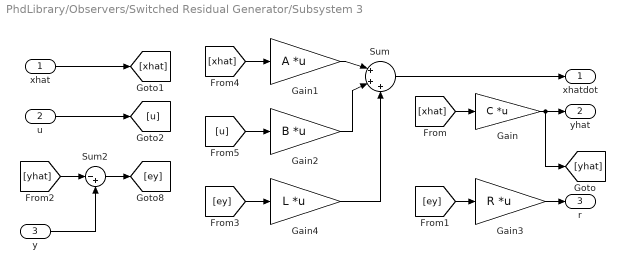
== system PhdLibrary/Observers/Switched Residual Generator/Subsystem 3 ==
  xhat : Inport
  u : Inport  Port=2
  y : Inport  Port=3
  Gain : Gain  Gain=C  Multiplication=Matrix(K*u) (u vector)
  Gain1 : Gain  Gain=A  Multiplication=Matrix(K*u) (u vector)
  Gain2 : Gain  Gain=B  Multiplication=Matrix(K*u) (u vector)
  Gain3 : Gain  Gain=R  Multiplication=Matrix(K*u) (u vector)
  Gain4 : Gain  Gain=L  Multiplication=Matrix(K*u) (u vector)
  Sum : Sum  Inputs=|+++
  Sum2 : Sum  Inputs=|-+
  xhatdot : Outport
  yhat : Outport  Port=2
  r : Outport  Port=3
  wires:
  Sum2/1 -> [ey]
  [yhat] -> Sum2/1
  y/1 -> Sum2/2
  Sum/1 -> xhatdot/1
  Gain/1 -> yhat/1, [yhat]
  xhat/1 -> [xhat]
  [xhat] -> Gain/1
  [ey] -> Gain3/1
  Gain3/1 -> r/1
  u/1 -> [u]
  [xhat] -> Gain1/1
  Gain1/1 -> Sum/1
  [u] -> Gain2/1
  Gain2/1 -> Sum/2
  Gain4/1 -> Sum/3
  [ey] -> Gain4/1

== system PhdLibrary/Observers/Uncertain Cuk/Subsystem ==
  x : Inport
  u : Inport  Port=2
  Gain : Gain  Gain=B  Multiplication=Matrix(K*u) (u vector)
  Gain1 : Gain  Gain=A  Multiplication=Matrix(K*u) (u vector)
  Gain2 : Gain  Gain=C  Multiplication=Matrix(K*u) (u vector)
  Sum : Sum  Inputs=|++
  xdot : Outport
  y : Outport  Port=2
  wires:
  u/1 -> Gain/1
  x/1 -> Gain2/1, Gain1/1
  Gain1/1 -> Sum/1
  Gain/1 -> Sum/2
  Sum/1 -> xdot/1
  Gain2/1 -> y/1

== system PhdLibrary/Observers/Uncertain Cuk/Subsystem1 ==
  x : Inport
  u : Inport  Port=2
  Gain : Gain  Gain=B  Multiplication=Matrix(K*u) (u vector)
  Gain1 : Gain  Gain=A  Multiplication=Matrix(K*u) (u vector)
  Gain2 : Gain  Gain=C  Multiplication=Matrix(K*u) (u vector)
  Sum : Sum  Inputs=|++
  xdot : Outport
  y : Outport  Port=2
  wires:
  u/1 -> Gain/1
  x/1 -> Gain2/1, Gain1/1
  Gain1/1 -> Sum/1
  Gain/1 -> Sum/2
  Sum/1 -> xdot/1
  Gain2/1 -> y/1

== system PhdLibrary/Controllers/Integral Sliding Mode Controller/SlidingSurface/If Action Subsystem ==
  S : Inport
  Action Port : ActionPort
  Sign : Signum
  d : Outport
  wires:
  S/1 -> Sign/1
  Sign/1 -> d/1

== system PhdLibrary/Controllers/Integral Sliding Mode Controller/SlidingSurface/If Action Subsystem2 ==
  S : Inport
  ep : Inport  Port=2
  Action Port : ActionPort
  Divide : Product  Inputs=*/
  d : Outport
  wires:
  S/1 -> Divide/1
  ep/1 -> Divide/2
  Divide/1 -> d/1

== system PhdLibrary/Observers/FDSMOSLS/ErrorGenerator/If Action Subsystem ==
  e_y : Inport
  Action Port : ActionPort
  Matrix Multiply : Product  Multiplication=Matrix(*)
  Matrix Multiply1 : Product
  Matrizes A1 : Constant  Value=rho
  Matrizes A2 : Constant  Value=F  VectorParams1D=off
  Normalization : dspmathops/Normalization  NormType=2-norm  Bias=1e-10  NormOver=Each column  Dimension=1  roundingMode=Floor  overflowMode=off  accumDataTypeStr=Inherit: Same as product output  accumLastDataTypeStr=Inherit: Same as product output  outputDataTypeStr=Inherit: Same as product output  outputMin=[]  outputMax=[]  outputLastDataTypeStr=Inherit: Same as product output
  v : Outport
  wires:
  Matrix Multiply1/1 -> v/1
  Matrizes A1/1 -> Matrix Multiply1/1
  e_y/1 -> Matrix Multiply/2
  Normalization/1 -> Matrix Multiply1/2
  Matrizes A2/1 -> Matrix Multiply/1
  Matrix Multiply/1 -> Normalization/1

== system PhdLibrary/Observers/FDSMOSLS/ErrorGenerator/If Action Subsystem1 ==
  e_y : Inport
  Action Port : ActionPort
  v : Outport
  wires:
  e_y/1 -> v/1

== system PhdLibrary/Observers/FDSMOSLS/Sliding Mode Observer 5/ObserverDynamics ==
  ey : Inport
  v : Inport  Port=2
  sigma : Inport  Port=3
  Gain : Gain  Gain=Atilde1  Multiplication=Matrix(K*u)
  Gain1 : Gain  Gain=G  Multiplication=Matrix(K*u)
  Gain3 : Gain  Gain=Dtilde1  Multiplication=Matrix(K*u)
  Gain5 : Gain  Gain=Atilde2  Multiplication=Matrix(K*u)
  Gain7 : Gain  Gain=Dtilde2  Multiplication=Matrix(K*u)
  Integral : Subsystem
  Sum : Sum  Inputs=|+++
  Sum1 : Sum  Inputs=|+++
  Switch1 : Switch  Criteria=u2 > Threshold
  e_tilde_hat : Outport
  wires:
  Gain/1 -> Sum/3
  Gain1/1 -> Sum/2, Sum1/1
  Gain3/1 -> Sum/1
  Gain5/1 -> Sum1/3
  Gain7/1 -> Sum1/2
  Sum/1 -> Switch1/1
  Sum1/1 -> Switch1/3
  v/1 -> Gain3/1, Gain7/1
  ey/1 -> Gain1/1
  Integral/1(e_hat) -> Gain5/1, e_tilde_hat/1, Gain/1
  Switch1/1 -> Integral/1(e_hat_dot)  "v"
  sigma/1 -> Switch1/2

== system PhdLibrary/Observers/FDSMOSLS/Sliding Mode Observer 5/ObserverDynamics/Integral ==
  e_hat_dot : Inport
  Ground{1..4} (4 alike) : Ground
  IC : InitialCondition  Value=[-xe;0;0]
  Integrator5 : Integrator  InitialConditionSource=external  InitialCondition=[-x_e; 0; 0]
  Mux : Mux
  e_hat : Outport
  wires:
  Mux/1 -> IC/1
  Ground4/1 -> Mux/4
  Ground3/1 -> Mux/3
  Ground2/1 -> Mux/2
  Ground1/1 -> Mux/1
  IC/1 -> Integrator5/2
  Integrator5/1 -> e_hat/1
  e_hat_dot/1 -> Integrator5/1

== matlab function PhdLibrary/Norms/Norm/Nom ==
  data: u input; y output
function y = fcn(u)

y = norm(u);
